simulink model "problem1Simulink"  (R2023a)
settings: Solver=VariableStepAuto  StartTime=0.0  StopTime=100  RelTol=1e-3
undefined symbols (not defined in the file): A, an, beta, Cd, Cr, g, m, rho, sgn, theta, Tm, wm
settings Model: Creator=rainsball  LastModifiedBy=rainsball

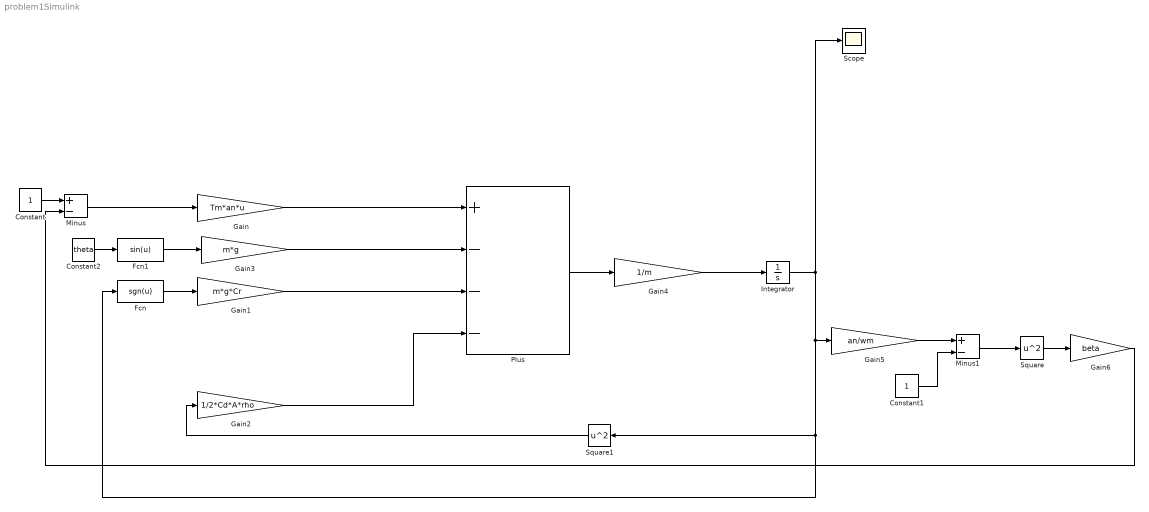
== system problem1Simulink ==
  Constant : Constant
  Constant1 : Constant
  Constant2 : Constant  Value=theta
  Fcn : Fcn  Expr=sgn(u)
  Fcn1 : Fcn  Expr=sin(u)
  Gain : Gain  Gain=Tm*an*u
  Gain1 : Gain  Gain=m*g*Cr
  Gain2 : Gain  Gain=1/2*Cd*A*rho
  Gain3 : Gain  Gain=m*g
  Gain4 : Gain  Gain=1/m
  Gain5 : Gain  Gain=an/wm
  Gain6 : Gain  Gain=beta
  Integrator : Integrator
  Minus : Sum  Inputs=+-
  Minus1 : Sum  Inputs=+-
  Plus : Sum  Inputs=+---
  Scope : Scope
  Square : Math  Operator=square
  Square1 : Math  Operator=square
  wires:
  Constant/1 -> Minus/1
  Minus/1 -> Gain/1
  Gain/1 -> Plus/1
  Gain1/1 -> Plus/3
  Plus/1 -> Gain4/1
  Gain4/1 -> Integrator/1
  Integrator/1 -> Square1/1, Fcn/1, Gain5/1, Scope/1
  Gain5/1 -> Minus1/1
  Constant1/1 -> Minus1/2
  Fcn/1 -> Gain1/1
  Gain2/1 -> Plus/4
  Gain3/1 -> Plus/2
  Fcn1/1 -> Gain3/1
  Constant2/1 -> Fcn1/1
  Minus1/1 -> Square/1
  Square/1 -> Gain6/1
  Gain6/1 -> Minus/2
  Square1/1 -> Gain2/1
